simulink model "CAVE_MachE_Testing_testing_V2"  (R2024a)
settings: configuration reference "ConfigSetDesktopFixedStep" (kept outside this file)
PreLoadFcn:
  | VSS_BICYCLE=Simulink.Variant('Dual=0');
  | VSS_DUAL=Simulink.Variant('Dual=1');
  | Dual=1;
  | load('DriveCycle2.mat')
PostLoadFcn:
  | if any(exist('dsrtsu_mdlpostloadfcn', 'file') ~= 0), dsrtsu_mdlpostloadfcn('Execute', bdroot); end
InitFcn:
  | , if any(exist('rtifpga_mdlclblib', 'file') ~= 0), rtifpga_mdlclblib('Init', bdroot); end,
  | , if any(exist('dsmpb_private', 'file') ~= 0), dsmpb_private('dsmpb_mdlclblib', 'Init', bdroot); end,
  | load('DriveCycle2.mat')
model workspace (MAT data in the model file):
  Gas = 0.383333333333
undefined symbols (not defined in the file or in its folder): AccelCmd, ActTqLF_Nm_, ActTqLR_Nm_, ActTqRF_Nm_, ActTqRR_Nm_, BattChargeLimitMaxPwr, BattChargeLimitSocBpts, BattChargeLimitTbl, BattChrgCapcty, BattDischargeLimitSocBpts, BattDischargeLimitTbl, BattDischargeMaxPwr, BattNumCellsParallel, BattNumCellsSeries, BattOpenVoltCapBpts, BattOpenVoltTbl, BattResistSocBpts, BattResistTbl, BattResistTempBpts, BrakeMaxPrs, BrakeMaxTrq, ChassisDistCg2FrontAxle, ChassisDistCg2RearAxle, ChassisVehMass, CltchCmd, CoastDown, DecelCmd, DiffRatio, DiscIntNeverNeededParam, EnvGravCnst, EnvPrs, EnvTemp, FuelSpecificGrav, GearCmd, h, InitStates, lgSw, limitedMCT, MCT, MtrEffSpdBpts, MtrEffTbl, MtrEffTrqBpts, MtrPwrMax, MtrTrqMax, out_1, pMCT, RealSimPara, Ref_speed, Ref_time, SteeringCmd, SupvsryCtrlRegenBrkCutOffTbl, SupvsryCtrlRegenSpdBpts, TestScnrioCycleNum, US06, VEH
libraries: VSIGenLib x65, simulink x54, etargetslib x38, dsmpblib x24, vehdynlibtire x12, autolibshared x11, vehdynlibsuspension x7, vehdynlibtirecommon x7, autolibpowerinfoutils x6, autolibutils x5, autolibsharedcoupling x4, autolibmappedmotor x4
(part 3 of 17)

== system CAVE_MachE_Testing_testing_V2/RealSim2/ToRealSim/RealSim CreatBus ==
  In : Inport
  speedDesired : Inport  Port=2
  color : Inport  Port=3
  accelerationDesired : Inport  Port=4
  activeLaneChange : Inport  Port=5
  Bus Creator2 : BusCreator  Inputs=36  OutDataTypeStr=Bus: VehDataBus
  Bus Selector1 : BusSelector  OutputSignals=id,idLength,type,typeLength,vehicleClass,vehicleClassLength,speed,acceleration,positionX,positionY,positionZ,heading,color,linkId,linkIdLength,laneId,distanceTravel,speedDesired,accelerationDesired,hasPrecedingVehicle,precedingVehicleId,precedingVehicleIdLength,precedingVehicleDistance,precedingVehicleSpeed,signalLightId,signalLightIdLength,signalLightHeadId,signalLightDistance,signalLightColor,speedLimit,speedLimitNext,speedLimitChangeDistance,linkIdNext,linkIdNextLength,grade,activeLaneChange
  Terminator{4..7} (4 alike) : Terminator
  rgba2uint : Subsystem
  Out : Outport
  wires:
  Bus Creator2/1 -> Out/1
  rgba2uint/1(Out1) -> Bus Creator2/13  "color"
  color/1 -> rgba2uint/1(In1)  "color"
  accelerationDesired/1 -> Bus Creator2/19  "accelerationDesired"
  speedDesired/1 -> Bus Creator2/18  "speedDesired"
  activeLaneChange/1 -> Bus Creator2/36  "activeLaneChange"
  Bus Selector1/36 -> Terminator7/1  "<activeLaneChange>"
  Bus Selector1/35 -> Bus Creator2/35  "<grade>"
  Bus Selector1/34 -> Bus Creator2/34  "<linkIdNextLength>"
  Bus Selector1/33 -> Bus Creator2/33  "<linkIdNext>"
  Bus Selector1/32 -> Bus Creator2/32  "<speedLimitChangeDistance>"
  Bus Selector1/31 -> Bus Creator2/31  "<speedLimitNext>"
  Bus Selector1/30 -> Bus Creator2/30  "<speedLimit>"
  Bus Selector1/29 -> Bus Creator2/29  "<signalLightColor>"
  Bus Selector1/28 -> Bus Creator2/28  "<signalLightDistance>"
  Bus Selector1/27 -> Bus Creator2/27  "<signalLightHeadId>"
  Bus Selector1/26 -> Bus Creator2/26  "<signalLightIdLength>"
  Bus Selector1/25 -> Bus Creator2/25  "<signalLightId>"
  Bus Selector1/24 -> Bus Creator2/24  "<precedingVehicleSpeed>"
  Bus Selector1/23 -> Bus Creator2/23  "<precedingVehicleDistance>"
  Bus Selector1/22 -> Bus Creator2/22  "<precedingVehicleIdLength>"
  Bus Selector1/21 -> Bus Creator2/21  "<precedingVehicleId>"
  Bus Selector1/20 -> Bus Creator2/20  "<hasPrecedingVehicle>"
  Bus Selector1/19 -> Terminator6/1  "<accelerationDesired>"
  Bus Selector1/18 -> Terminator4/1  "<speedDesired>"
  Bus Selector1/17 -> Bus Creator2/17  "<distanceTravel>"
  Bus Selector1/16 -> Bus Creator2/16  "<laneId>"
  Bus Selector1/15 -> Bus Creator2/15  "<linkIdLength>"
  Bus Selector1/14 -> Bus Creator2/14  "<linkId>"
  Bus Selector1/13 -> Terminator5/1  "<color>"
  Bus Selector1/12 -> Bus Creator2/12  "<heading>"
  Bus Selector1/11 -> Bus Creator2/11  "<positionZ>"
  Bus Selector1/10 -> Bus Creator2/10  "<positionY>"
  Bus Selector1/9 -> Bus Creator2/9  "<positionX>"
  Bus Selector1/8 -> Bus Creator2/8  "<acceleration>"
  Bus Selector1/7 -> Bus Creator2/7  "<speed>"
  Bus Selector1/6 -> Bus Creator2/6  "<vehicleClassLength>"
  Bus Selector1/5 -> Bus Creator2/5  "<vehicleClass>"
  Bus Selector1/4 -> Bus Creator2/4  "<typeLength>"
  Bus Selector1/3 -> Bus Creator2/3  "<type>"
  Bus Selector1/2 -> Bus Creator2/2  "<idLength>"
  Bus Selector1/1 -> Bus Creator2/1  "<id>"
  In/1 -> Bus Selector1/1

== system CAVE_MachE_Testing_testing_V2/Vehicle Under Test1/Environment/Ground Feedback ==
  note: 1) Add Subsystem or Model blocks as valid variant choices.
      | 2) You cannot connect blocks at this level. At simulation, connectivity is automatically
      | determined, based on the active variant and port name matching.
  Friction : Inport
  Ground Z Level : Inport  Port=2
  3D Engine : Subsystem  VariantControl=1
  Constant : Subsystem  VariantControl=0
  Ground : Outport  VectorParamsAs1DForOutWhenUnconnected=off

== system CAVE_MachE_Testing_testing_V2/Vehicle Under Test1/Environment/Subsystem ==
  Grade : Inport
  Constant : Constant  Value=EnvPrs
  Constant1 : Constant  Value=EnvTemp
  Constant2 : Constant  Value=0
  Constant3 : Constant  Value=0
  Constant4 : Constant  Value=0
  Signal Specification : SignalSpecification  Unit=Pa
  Signal Specification1 : SignalSpecification  Unit=K
  Signal Specification2 : SignalSpecification  Unit=rad
  Signal Specification3 : SignalSpecification  Unit=m/s
  Signal Specification4 : SignalSpecification  Unit=m/s
  Signal Specification5 : SignalSpecification  Unit=m/s
  Vector Concatenate : Concatenate  NumInputs=3
  EnvPrs : Outport
  EnvTemp : Outport  Port=2
  WindVel : Outport  Port=3
  RoadGrade : Outport  Port=4
  wires:
  Signal Specification5/1 -> Vector Concatenate/3  "WindZ"
  Signal Specification4/1 -> Vector Concatenate/2  "WindY"
  Constant4/1 -> Signal Specification5/1
  Constant3/1 -> Signal Specification4/1
  Signal Specification3/1 -> Vector Concatenate/1  "WindX"
  Vector Concatenate/1 -> WindVel/1
  Signal Specification2/1 -> RoadGrade/1
  Signal Specification1/1 -> EnvTemp/1
  Signal Specification/1 -> EnvPrs/1
  Grade/1 -> Signal Specification2/1
  Constant1/1 -> Signal Specification1/1
  Constant2/1 -> Signal Specification3/1
  Constant/1 -> Signal Specification/1

== system CAVE_MachE_Testing_testing_V2/Vehicle Under Test1/Environment/Subsystem1 ==
  EnvPrs : Inport
  EnvTemp : Inport  Port=2
  WindVel : Inport  Port=3
  RoadGrade : Inport  Port=4
  GroundBus : Inport  Port=5
  Bus Creator : BusCreator  Inputs=5
  Env : Outport
  wires:
  GroundBus/1 -> Bus Creator/5  "GndBus"
  RoadGrade/1 -> Bus Creator/4  "RoadGrade"
  WindVel/1 -> Bus Creator/3  "WindVel"
  Bus Creator/1 -> Env/1  "Env"
  EnvTemp/1 -> Bus Creator/2  "EnvTemp"
  EnvPrs/1 -> Bus Creator/1  "EnvPrs"

== system CAVE_MachE_Testing_testing_V2/Vehicle Under Test1/Monitor/Calculate Fuel MPG ==
  Monitor : Inport
  Bus Selector : BusSelector  OutputSignals=Veh.Chassis.VehDist,Veh.Batt.EngPlant.FuellMassFlw
  Constant : Constant  Value=FuelSpecificGrav
  Density of Water : Gain  Gain=997
  Divide : Product  Inputs=*/
  Divide1 : Product  Inputs=*/
  Integrator : Integrator
  Saturation : Saturate  UpperLimit=inf  LowerLimit=1e-7
  Signal Specification : SignalSpecification  Unit=mi
  Signal Specification1 : SignalSpecification  Unit=m^3
  Signal Specification2 : SignalSpecification  Unit=gal
  Unit Conversion : UnitConversion
  Unit Conversion1 : UnitConversion
  FuelEconMPG : Outport
  wires:
  Signal Specification/1 -> Divide1/1  "VehDistMiles"
  Monitor/1 -> Bus Selector/1
  Signal Specification1/1 -> Unit Conversion1/1
  Constant/1 -> Density of Water/1
  Saturation/1 -> Divide1/2  "FuelVolume"
  Density of Water/1 -> Divide/2
  Integrator/1 -> Divide/1  "FuelMass"
  Bus Selector/2 -> Integrator/1  "<FuellMassFlw>"
  Bus Selector/1 -> Unit Conversion/1  "<VehDist>"
  Unit Conversion/1 -> Signal Specification/1
  Signal Specification2/1 -> Saturation/1
  Unit Conversion1/1 -> Signal Specification2/1
  Divide/1 -> Signal Specification1/1
  Divide1/1 -> FuelEconMPG/1  "FuelEconMPG"

== system CAVE_MachE_Testing_testing_V2/Vehicle Under Test1/Monitor/Calculate Powertrain Energy ==
  Monitor : Inport
  Bus Selector2 : BusSelector  OutputSignals=Veh.Diff.PwrInfo.PwrTrnsfrd.PwrTrnsfrd.PwrDriveshft
  Integrator : Integrator
  Signal Specification : SignalSpecification  Unit=J
  Signal Specification1 : SignalSpecification  Unit=kW*h
  Unit Conversion : UnitConversion
  TransEnrgyOutkWh : Outport
  wires:
  Bus Selector2/1 -> Integrator/1  "<PwrDriveshft>"
  Monitor/1 -> Bus Selector2/1
  Signal Specification1/1 -> TransEnrgyOutkWh/1
  Signal Specification/1 -> Unit Conversion/1
  Integrator/1 -> Signal Specification/1  "EnrgyTrans"
  Unit Conversion/1 -> Signal Specification1/1

== system CAVE_MachE_Testing_testing_V2/Vehicle Under Test1/Vehicle/Actuation and Outputs ==
  note: Driver Commands are [0,100] for both pedal and brake
  Driver Commands : Inport
  CarlaGBS : Inport  Port=2
  APP : Constant  Value=0
  AR_limit : Saturate  UpperLimit=65  LowerLimit=0
  BR_command_0to100 : Constant  Value=0
  BR_limit : Saturate  UpperLimit=70  LowerLimit=0
  Bus Creator : BusCreator  Inputs=2
  Bus Selector1 : BusSelector  OutputSignals=AccelPedalCmd
  Bus Selector3 : BusSelector  OutputSignals=BrakePedalCmd
  Constant : Constant  Value=0
  Constant1 : Constant  Value=0
  Demux : Demux  Outputs=3
  Gain : Gain  Gain=100
  Gain1 : Gain  Gain=100
  MOOG Brake Actuator : Subsystem
  Min threshold for Brake switch : Constant  Value=0
  Multiport Switch1 : MultiPortSwitch  Inputs=4  SaturateOnIntegerOverflow=off  InputSameDT=off
  Multiport Switch2 : MultiPortSwitch  Inputs=4  SaturateOnIntegerOverflow=off  InputSameDT=off
  Pedal Robot Control Selection : Constant  Value=2
  Relational Operator : RelationalOperator  Operator=>  OutDataTypeStr=boolean  InputSameDT=off
  Scope1 : Scope  NumInputPorts=2
  Vehicle Accel Pedal Voltage Output : Subsystem
  bped2br_N : Lookup_n-D  NumberOfTableDimensions=1  BreakpointsForDimension1=[0 0.1 0.2 100]  Table=[0 0 25 100]  InternalRulePriority=Speed  RndMeth=Simplest
  BrakeSwitch : Outport  VectorParamsAs1DForOutWhenUnconnected=off
  CAVE_Driver : Outport  Port=2
  tag scope: BrakeDriver=global, CarlaSteer=global, GasDriver=global
  wires:
  [BrakeDriver] -> Scope1/2
  [GasDriver] -> Scope1/1
  Demux/3 -> [CarlaSteer]
  Gain1/1 -> Multiport Switch2/4
  Gain/1 -> Multiport Switch1/4
  CarlaGBS/1 -> Demux/1
  Demux/2 -> Gain1/1
  Demux/1 -> Gain/1
  BR_limit/1 -> bped2br_N/1, Relational Operator/1, Bus Creator/2, [BrakeDriver]  "BrakePedalCmd_pct"
  AR_limit/1 -> Vehicle Accel Pedal Voltage Output/1(APP_pct), Bus Creator/1, [GasDriver]  "AccelPedalCmd_pct"
  Bus Creator/1 -> CAVE_Driver/1
  Constant1/1 -> Multiport Switch2/5
  Constant/1 -> Multiport Switch1/5
  Relational Operator/1 -> BrakeSwitch/1  "BrakeSwitch"
  Min threshold for Brake switch/1 -> Relational Operator/2
  bped2br_N/1 -> MOOG Brake Actuator/1(Brake Pedal command [%])
  Bus Selector3/1 -> Multiport Switch2/3  "<BrakePedalCmd>"
  BR_command_0to100/1 -> Multiport Switch2/2
  Pedal Robot Control Selection/1 -> Multiport Switch2/1, Multiport Switch1/1
  Driver Commands/1 -> Bus Selector1/1, Bus Selector3/1
  Multiport Switch2/1 -> BR_limit/1
  Bus Selector1/1 -> Multiport Switch1/3  "<AccelPedalCmd>"
  APP/1 -> Multiport Switch1/2
  Multiport Switch1/1 -> AR_limit/1

== system CAVE_MachE_Testing_testing_V2/Vehicle Under Test1/Vehicle/Battery ==
  Battery : Subsystem
  Subsystem1 : Subsystem
      mask Display: disp('')
  BattOut : PMIOPort  Side=Right
  BattOut1 : PMIOPort  Port=2  Side=Right
  Batt : Outport
  wires:
  Subsystem1/1(Batt) -> Batt/1
  Battery/3(BattVolt) -> Subsystem1/3(BattVolt)
  Battery/2(BattCurr) -> Subsystem1/2(BattCurr)
  Battery/1(BattSoc) -> Subsystem1/1(BattSoc)
  connections:
  BattOut/RConn1 -- Battery/RConn1
  Battery/RConn2 -- BattOut1/RConn1

== system CAVE_MachE_Testing_testing_V2/Vehicle Under Test1/Vehicle/Driver and Drive Cycle ==
  Veh speed feedback [kph] : Inport
  Veh speed cycle trigger : Inport  Port=2
  SUMO Veh speed Cmd Level : Inport  Port=3
  CarlaRef : Inport  Port=4
  1-D Lookup Table : Lookup_n-D  NumberOfTableDimensions=1  BreakpointsForDimension1=Ref_time  Table=Ref_speed  InternalRulePriority=Speed  RndMeth=Simplest
  Add : Sum
  Add1 : Sum  Inputs=+-
  Add2 : Sum
  Clock : Clock
  Clock1 : Clock
  CoastDown : Lookup_n-D  Commented=on  NumberOfTableDimensions=1  BreakpointsForDimension1=CoastDown.Time  Table=CoastDown.Speed  InternalRulePriority=Speed  RndMeth=Simplest
  Constant : Constant  Value=0
  Data Type Conversion11 : DataTypeConversion  OutDataTypeStr=double  SaturateOnIntegerOverflow=off  RndMeth=Floor  LockScale=on
  Demux : Demux  Outputs=3
  DriveCycleSelect : Constant  Commented=on
  Driver and PI with FF Control : Subsystem
  Gain : Gain  Gain=1/1.609
  Gain1 : Gain  Gain=1/1.609
  Gain2 : Gain  Gain=3.6
  Gain3 : Gain  Gain=3.6
  Get Cycle Clock Time : Subsystem
  MCT : Lookup_n-D  Commented=on  NumberOfTableDimensions=1  BreakpointsForDimension1=MCT.Time  Table=MCT.Speed  InternalRulePriority=Speed  RndMeth=Simplest
  ManSpd : Constant  Value=0
  ManSpdSel1 : Constant  Value=2
  Memory4 : Memory
  Multiport Switch : MultiPortSwitch  Commented=on  Inputs=5  SaturateOnIntegerOverflow=off  InputSameDT=off
  Multiport Switch1 : MultiPortSwitch  Inputs=4  SaturateOnIntegerOverflow=off  InputSameDT=off
  Rate Limiter : RateLimiter  RisingSlewLimit=5  FallingSlewLimit=-5  SampleTimeMode=inherited
  Scope : Scope  NumInputPorts=2
  Switch1 : Switch  Threshold=3  SaturateOnIntegerOverflow=off  InputSameDT=off
  Terminator{,1..3} (4 alike) : Terminator
  Terminator4 : Terminator  Commented=on
  US06 : Lookup_n-D  Commented=on  NumberOfTableDimensions=1  BreakpointsForDimension1=US06.Time  Table=US06.Speed  InternalRulePriority=Speed  RndMeth=Simplest
  US1 : Lookup_n-D  NumberOfTableDimensions=1  BreakpointsForDimension1=US06.Time  Table=US06.Speed  InternalRulePriority=Speed  RndMeth=Simplest
  driver look ahead seconds : Constant  Value=0.5
  limitedMCT : Lookup_n-D  Commented=on  NumberOfTableDimensions=1  BreakpointsForDimension1=limitedMCT.Time  Table=limitedMCT.Speed  InternalRulePriority=Speed  RndMeth=Simplest
  pMCT : Lookup_n-D  Commented=on  NumberOfTableDimensions=1  BreakpointsForDimension1=pMCT.Time  Table=pMCT.Speed  InternalRulePriority=Speed  RndMeth=Simplest
  DriverBus : Outport
  ManSpdSel : Outport  Port=2
  wires:
  US1/1 -> Rate Limiter/1
  Clock/1 -> Switch1/3
  Add2/1 -> Gain3/1
  Gain3/1 -> Multiport Switch1/4
  Memory4/1 -> Switch1/1
  Switch1/1 -> Memory4/1, Add1/2
  SUMO Veh speed Cmd Level/1 -> Add2/2
  Add1/1 -> 1-D Lookup Table/1  "tCycle"
  1-D Lookup Table/1 -> Add2/1
  ManSpdSel1/1 -> ManSpdSel/1, Multiport Switch1/1, Switch1/2
  Clock1/1 -> Add1/1, US1/1
  Constant/1 -> Multiport Switch1/5
  Demux/3 -> Terminator3/1
  Demux/2 -> Terminator2/1
  Demux/1 -> Gain2/1
  CarlaRef/1 -> Demux/1
  Gain2/1 -> Multiport Switch1/3
  Multiport Switch/1 -> Terminator4/1
  Rate Limiter/1 -> Multiport Switch1/2
  Multiport Switch1/1 -> Driver and PI with FF Control/2(Vehicle_SpdDmd_kph), Gain1/1, Scope/2  "RefSpd [km/hr]"
  Gain1/1 -> Terminator1/1  "Vehicle_SpdDmd_mph"
  Gain/1 -> Terminator/1  "Vehicle_Spd_mph"
  Veh speed feedback [kph]/1 -> [VehSpdKph]
  limitedMCT/1 -> Multiport Switch/6
  driver look ahead seconds/1 -> Add/1
  Get Cycle Clock Time/1(tCycle) -> Add/2
  Data Type Conversion11/1 -> Driver and PI with FF Control/1(Vehicle_Spd_kph), Scope/1, Gain/1  "Vehicle_Spd_kph"
  Driver and PI with FF Control/1(DriverBus) -> DriverBus/1
  [VehSpdKph] -> Data Type Conversion11/1
  DriveCycleSelect/1 -> Multiport Switch/1
  pMCT/1 -> Multiport Switch/3
  CoastDown/1 -> Multiport Switch/2
  Add/1 -> US06/1, MCT/1, limitedMCT/1, pMCT/1, CoastDown/1
  US06/1 -> Multiport Switch/4
  MCT/1 -> Multiport Switch/5
  Veh speed cycle trigger/1 -> Get Cycle Clock Time/1(Cycle Trigger)

== system CAVE_MachE_Testing_testing_V2/Vehicle Under Test1/Vehicle/From CAN ==
  BrakeSwitch : Inport
  Brake switch ource selection : Constant  Value=2
  Bus Creator1 : BusCreator  Inputs=2
  Demux : Demux  Outputs=1
  Ground : Ground
  Ground1 : Ground
  Multiport Switch1 : MultiPortSwitch  Inputs=2  SaturateOnIntegerOverflow=off  InputSameDT=off
  IO_Out : Outport
  wires:
  BrakeSwitch/1 -> Multiport Switch1/3
  Ground1/1 -> Multiport Switch1/2  "Brake switch from CAN"
  Brake switch ource selection/1 -> Multiport Switch1/1
  Ground/1 -> Demux/1
  Demux/1 -> Bus Creator1/1  "STEERING_ANGLE_DEG_CAN"
  Multiport Switch1/1 -> Bus Creator1/2  "BRAKE_LAMP_BOOL_CAN"
  Bus Creator1/1 -> IO_Out/1  "IO_Out"

== system CAVE_MachE_Testing_testing_V2/Vehicle Under Test1/Vehicle/Front Wheel Drive ==
  DrvShfTrq : Inport
  Omega : Inport  Port=2
  Ideal Diff : Subsystem  VariantControl=0
  Ideal Diff AWD : Subsystem  VariantControl=Choice
  Real Diff : Subsystem  VariantControl=1
  Diff : Outport  VectorParamsAs1DForOutWhenUnconnected=off
  AxlTrq : Outport  Port=2  VectorParamsAs1DForOutWhenUnconnected=off
  PropShaftSpd : Outport  Port=3  VectorParamsAs1DForOutWhenUnconnected=off
  PropShaftSpd1 : Outport  Port=4

== system CAVE_MachE_Testing_testing_V2/Vehicle Under Test1/Vehicle/Motor_F ==
  SupvsryCtrl : Inport
  MtrSpd : Inport  Port=2
  Bus Creator1 : BusCreator  Inputs=1
  Bus Creator2 : BusCreator  Inputs=4
  Bus Selector1 : BusSelector  OutputSignals=Volt
  Bus Selector2 : BusSelector  OutputSignals=MtrTrqCmd
  Bus Selector3 : BusSelector  OutputSignals=PwrInfo.PwrTrnsfrd.PwrMtr,PwrInfo.PwrTrnsfrd.PwrBus
  Mach-E Motor : autolibmappedmotor/Mapped Motor  port_config=Speed  param_by=Maximum torque and power  w_t=[ 0 375 750 800 ]  T_t=[0.09 0.08 0.07 0]  torque_max=800  power_max=358000  Tc=0.01  param_loss=Tabulated efficiency data  eff=100  w_eff=375  T_eff=0.08  Piron=0  Pbase=0  w_eff_bp=MtrEffSpdBpts.*pi/30  T_eff_bp=MtrEffTrqBpts  Temp_eff_bp=[233.15 293.15 373.15]  losses_table=[1 2;3 4]  losses_table_3d=cat(3,[1.49 1.67 2.21 3.10; 0.42 0.69 1.14 2.03; 0.06 0.24 0.78 1.68; 0.42 0.69 1.14 2.03; 1.49 1.67 2.21 3.10],[1.49 1.67 2.21 3.10; 0.42 0.69 1.14 2.03; 0.06 0.24 0.78 1.68; 0.42 0.69 1.14 2.03; 1.49 1.67 2.21 3.10],[1.49 1.67 2.21 3.10; 0.42 0.69 1.14 2.03; 0.06 0.24 0.78 1.68; 0.42 0.69 1.14 2.03; 1.49 1.67 2.21 3.10])  efficiency_table=MtrEffTbl*0.94  efficiency_table_3d=cat(3,[95 95 95 95; 95 95 95 95; 95 95 95 95; 95 95 95 95; 95 95 95 95],[95 95 95 95; 95 95 95 95; 95 95 95 95; 95 95 95 95; 95 95 95 95],[95 95 95 95; 95 95 95 95; 95 95 95 95; 95 95 95 95; 95 95 95 95])  J=5e-6  b=1e-5  omega_o=0  T_t_extended=[0 0.07 0.08 0.09 0.08 0.07 0]  w_t_extended=[-800 -750 -375 0 375 750 800]  KLossIron=0  KLossCopper=0  x_w_eff_vec=[-1047.1975511966 -942.477796076938 -837.758040957278 -733.038285837618 -628.318530717959 -523.598775598299 -418.879020478639 -314.159265358979 -285.714285713875 -209.43951023932 -104.71975511966 0 104.71975511966 209.43951023932 285.714285713875 314.159265358979 418.879020478639 523.598775598299 628.318530717959 733.038285837618 837.758040957278 942.477796076938 1047.1975511966]  x_T_eff_vec=[-360 -334.285714285714 -308.571428571429 -282.857142857143 -257.142857142857 -231.428571428571 -205.714285714286 -180 -154.285714285714 -128.571428571429 -102.857142857143 -77.1428571428572 -51.4285714285714 -25.7142857142857 0 25.7142857142857 51.4285714285714 77.1428571428572 102.857142857143 128.571428571429 154.285714285714 180 205.714285714286 231.428571428571 257.142857142857 282.857142857143 308.571428571429 334.285714285714 360]  x_tmp_eff_vec=[-0.09 -0.06 -0.03 0 0.03 0.06 0.09]  x_losses_mat=[54250.1517943165 50375.1409518653 46500.1301094142 42625.119266963 38750.1084245118 34875.0975820605 31000.0867396095 27125.0758971582 23250.065054707 19375.054212256 15500.0433698047 12629.4764797412 9803.55154311708 6774.11181875432 0 5412.5153431847 8293.80460547705 10921.9712596802 13550.1379138833 16937.6723923542 20325.2068708249 23712.7413492957 27100.2758277666 30487.8103062373 33875.3447847082 37262.879263179 40650.4137416499 44037.9482201206 47425.4826985915;44696.230836134 41503.6429192672 38311.0550024006 35118.4670855338 31925.8791686671 28733.2912518003 25540.7033349337 22348.115418067 19155.5275012002 15962.9395843336 12770.3516674669 9577.76375060014 6975.01951641212 6096.70063687888 0 4871.26380886623 6097.56206124747 8462.91205003029 11283.8827333737 14104.8534167172 16925.8241000605 19746.794783404 22567.7654667475 25388.7361500908 28209.7068334343 31030.6775167777 33851.6482001212 36672.6188834645 39493.589566808;36137.1105685043 33555.8883850397 30974.6662015752 28393.4440181105 25812.2218346459 23230.9996511813 20649.7774677168 18068.5552842522 15487.3331007875 12906.110917323 10324.8887338584 8513.56777831124 6200.01734792188 5419.28945500345 0 4330.01227454776 5420.05516555331 7522.58848891581 9220.12563933554 11525.1570491694 13830.1884590033 16135.2198688372 18440.2512786711 20745.2826885049 23050.3140983388 25355.3455081727 27660.3769180066 29965.4083278404 32270.4397376744;31619.9717474413 29361.4023369097 27102.8329263783 24844.2635158467 22585.6941053152 20327.1246947836 18068.5552842522 15809.9858737206 13551.4164631891 11292.8470526576 9034.27764212609 7449.37180602233 5425.01517943165 4741.87827312802 0 3788.76074022929 4742.54826985915 6582.26492780134 8067.6099344186 10084.5124180233 12101.4149016279 14118.3173852325 16135.2198688372 18152.1223524418 20169.0248360465 22185.9273196511 24202.8298032558 26219.7322868604 28236.6347704651;27102.8329263782 25166.9162887798 23230.9996511814 21295.0830135829 19359.1663759844 17423.249738386 15487.3331007876 13551.4164631891 11615.4998255906 9679.58318799226 8513.56777831124 6385.17583373343 4650.01301094141 4064.46709125259 0 3247.50920591082 4065.04137416498 5641.94136668686 7522.58848891582 8643.86778687709 10372.6413442524 12101.4149016279 13830.1884590033 15558.9620163787 17287.7355737541 19016.5091311295 20745.282688505 22474.0562458803 24202.8298032558;22585.6941053152 20972.4302406498 19359.1663759845 17745.9025113191 16132.6386466537 14519.3747819883 12906.110917323 11292.8470526576 9679.58318799221 8066.31932332688 7094.63981525937 5320.97986144452 3875.01084245118 3387.05590937716 0 2706.25767159235 3387.53447847082 4701.61780557238 6268.82374076318 7203.22315573091 8643.86778687704 10084.5124180232 11525.1570491694 12965.8016803156 14406.4463114618 15847.0909426079 17287.7355737541 18728.3802049003 20169.0248360465;19864.9914827262 18446.0635196743 17027.1355566225 15608.2075935706 14189.2796305187 12770.3516674668 11351.423704415 9932.4957413631 8513.56777831121 7094.63981525938 5675.71185220749 4256.78388915562 3100.00867396094 2709.64472750173 0 2165.00613727388 2710.02758277665 3761.29424445791 5015.05899261055 6268.82374076319 7522.58848891579 8776.35323706844 10030.1179852211 11283.8827333737 12537.6474815263 13791.412229679 15045.1769778316 16298.9417259842 17552.7064741369;20587.4582405459 19116.9255090783 17646.3927776108 16175.8600461432 12629.4764797412 11366.528831767 10103.581183793 8137.52276914747 6975.01951641211 5812.51626367679 4650.01301094142 3788.84294392236 2525.89529594824 2032.23354562629 0 1623.75460295541 2184.39425193603 3276.59137790406 4065.04137416499 5081.30171770625 6097.56206124746 7113.82240478872 8737.57700774416 9829.77413371214 10921.9712596802 13684.7775990372 14928.8482898587 16172.9189806802 17416.9896715018;18723.4042552922 17386.0182370571 16048.6322188219 14711.2462005868 11485.9634880614 10337.3671392553 9188.77079044916 8040.174441643 6891.57809283685 5742.98174403074 4594.38539522458 ...(+6536 chars)]  x_losses_mat_3d=[37.8947368421052 25.2631578947368 12.6315789473684 0 12 24 36;18.9473684210526 12.6315789473684 6.3157894736842 0 5.99999999999999 12 18;0 0 0 0 0 0 0;18 12 5.99999999999999 0 6.3157894736842 12.6315789473684 18.9473684210526;36 24 12 0 12.6315789473684 25.2631578947368 37.8947368421052]  CalLossMapData={}  CalLossWithTempMapData={}  aMode=aMode  RefBlkName='autolibmappedmotor/Mapped Motor'
  Mapped Motor : autolibmappedmotor/Mapped Motor  port_config=Speed  param_by=Maximum torque and power  w_t=[ 0 375 750 800 ]  T_t=[0.09 0.08 0.07 0]  torque_max=MtrTrqMax  power_max=MtrPwrMax  Tc=MtrTrqTimeCnst  param_loss=Tabulated efficiency data  eff=100  w_eff=375  T_eff=0.08  Piron=0  Pbase=0  w_eff_bp=MtrEffSpdBpts.*pi/30  T_eff_bp=MtrEffTrqBpts  Temp_eff_bp=[233.15 293.15 373.15]  losses_table=[1 2;3 4]  losses_table_3d=cat(3,[1.49 1.67 2.21 3.10; 0.42 0.69 1.14 2.03; 0.06 0.24 0.78 1.68; 0.42 0.69 1.14 2.03; 1.49 1.67 2.21 3.10],[1.49 1.67 2.21 3.10; 0.42 0.69 1.14 2.03; 0.06 0.24 0.78 1.68; 0.42 0.69 1.14 2.03; 1.49 1.67 2.21 3.10],[1.49 1.67 2.21 3.10; 0.42 0.69 1.14 2.03; 0.06 0.24 0.78 1.68; 0.42 0.69 1.14 2.03; 1.49 1.67 2.21 3.10])  efficiency_table=MtrEffTbl*0.94  efficiency_table_3d=cat(3,[95 95 95 95; 95 95 95 95; 95 95 95 95; 95 95 95 95; 95 95 95 95],[95 95 95 95; 95 95 95 95; 95 95 95 95; 95 95 95 95; 95 95 95 95],[95 95 95 95; 95 95 95 95; 95 95 95 95; 95 95 95 95; 95 95 95 95])  J=5e-6  b=1e-5  omega_o=0  T_t_extended=[0 0.07 0.08 0.09 0.08 0.07 0]  w_t_extended=[-800 -750 -375 0 375 750 800]  KLossIron=0  KLossCopper=0  x_w_eff_vec=[-1047.1975511966 -942.477796076938 -837.758040957278 -733.038285837618 -628.318530717959 -523.598775598299 -418.879020478639 -314.159265358979 -285.714285713875 -209.43951023932 -104.71975511966 0 104.71975511966 209.43951023932 285.714285713875 314.159265358979 418.879020478639 523.598775598299 628.318530717959 733.038285837618 837.758040957278 942.477796076938 1047.1975511966]  x_T_eff_vec=[-360 -334.285714285714 -308.571428571429 -282.857142857143 -257.142857142857 -231.428571428571 -205.714285714286 -180 -154.285714285714 -128.571428571429 -102.857142857143 -77.1428571428572 -51.4285714285714 -25.7142857142857 0 25.7142857142857 51.4285714285714 77.1428571428572 102.857142857143 128.571428571429 154.285714285714 180 205.714285714286 231.428571428571 257.142857142857 282.857142857143 308.571428571429 334.285714285714 360]  x_tmp_eff_vec=[-0.09 -0.06 -0.03 0 0.03 0.06 0.09]  x_losses_mat=[54250.1517943165 50375.1409518653 46500.1301094142 42625.119266963 38750.1084245118 34875.0975820605 31000.0867396095 27125.0758971582 23250.065054707 19375.054212256 15500.0433698047 12629.4764797412 9803.55154311708 6774.11181875432 0 5412.5153431847 8293.80460547705 10921.9712596802 13550.1379138833 16937.6723923542 20325.2068708249 23712.7413492957 27100.2758277666 30487.8103062373 33875.3447847082 37262.879263179 40650.4137416499 44037.9482201206 47425.4826985915;44696.230836134 41503.6429192672 38311.0550024006 35118.4670855338 31925.8791686671 28733.2912518003 25540.7033349337 22348.115418067 19155.5275012002 15962.9395843336 12770.3516674669 9577.76375060014 6975.01951641212 6096.70063687888 0 4871.26380886623 6097.56206124747 8462.91205003029 11283.8827333737 14104.8534167172 16925.8241000605 19746.794783404 22567.7654667475 25388.7361500908 28209.7068334343 31030.6775167777 33851.6482001212 36672.6188834645 39493.589566808;36137.1105685043 33555.8883850397 30974.6662015752 28393.4440181105 25812.2218346459 23230.9996511813 20649.7774677168 18068.5552842522 15487.3331007875 12906.110917323 10324.8887338584 8513.56777831124 6200.01734792188 5419.28945500345 0 4330.01227454776 5420.05516555331 7522.58848891581 9220.12563933554 11525.1570491694 13830.1884590033 16135.2198688372 18440.2512786711 20745.2826885049 23050.3140983388 25355.3455081727 27660.3769180066 29965.4083278404 32270.4397376744;31619.9717474413 29361.4023369097 27102.8329263783 24844.2635158467 22585.6941053152 20327.1246947836 18068.5552842522 15809.9858737206 13551.4164631891 11292.8470526576 9034.27764212609 7449.37180602233 5425.01517943165 4741.87827312802 0 3788.76074022929 4742.54826985915 6582.26492780134 8067.6099344186 10084.5124180233 12101.4149016279 14118.3173852325 16135.2198688372 18152.1223524418 20169.0248360465 22185.9273196511 24202.8298032558 26219.7322868604 28236.6347704651;27102.8329263782 25166.9162887798 23230.9996511814 21295.0830135829 19359.1663759844 17423.249738386 15487.3331007876 13551.4164631891 11615.4998255906 9679.58318799226 8513.56777831124 6385.17583373343 4650.01301094141 4064.46709125259 0 3247.50920591082 4065.04137416498 5641.94136668686 7522.58848891582 8643.86778687709 10372.6413442524 12101.4149016279 13830.1884590033 15558.9620163787 17287.7355737541 19016.5091311295 20745.282688505 22474.0562458803 24202.8298032558;22585.6941053152 20972.4302406498 19359.1663759845 17745.9025113191 16132.6386466537 14519.3747819883 12906.110917323 11292.8470526576 9679.58318799221 8066.31932332688 7094.63981525937 5320.97986144452 3875.01084245118 3387.05590937716 0 2706.25767159235 3387.53447847082 4701.61780557238 6268.82374076318 7203.22315573091 8643.86778687704 10084.5124180232 11525.1570491694 12965.8016803156 14406.4463114618 15847.0909426079 17287.7355737541 18728.3802049003 20169.0248360465;19864.9914827262 18446.0635196743 17027.1355566225 15608.2075935706 14189.2796305187 12770.3516674668 11351.423704415 9932.4957413631 8513.56777831121 7094.63981525938 5675.71185220749 4256.78388915562 3100.00867396094 2709.64472750173 0 2165.00613727388 2710.02758277665 3761.29424445791 5015.05899261055 6268.82374076319 7522.58848891579 8776.35323706844 10030.1179852211 11283.8827333737 12537.6474815263 13791.412229679 15045.1769778316 16298.9417259842 17552.7064741369;20587.4582405459 19116.9255090783 17646.3927776108 16175.8600461432 12629.4764797412 11366.528831767 10103.581183793 8137.52276914747 6975.01951641211 5812.51626367679 4650.01301094142 3788.84294392236 2525.89529594824 2032.23354562629 0 1623.75460295541 2184.39425193603 3276.59137790406 4065.04137416499 5081.30171770625 6097.56206124746 7113.82240478872 8737.57700774416 9829.77413371214 10921.9712596802 13684.7775990372 14928.8482898587 16172.9189806802 17416.9896715018;18723.4042552922 17386.0182370571 16048.6322188219 14711.2462005868 11485.9634880614 10337.3671392553 9188.77079044916 8040.174441643 6891.57809283685 5742.98174403074 4594.38539522458 ...(+6536 chars)]  x_losses_mat_3d=[37.8947368421052 25.2631578947368 12.6315789473684 0 12 24 36;18.9473684210526 12.6315789473684 6.3157894736842 0 5.99999999999999 12 18;0 0 0 0 0 0 0;18 12 5.99999999999999 0 6.3157894736842 12.6315789473684 18.9473684210526;36 24 12 0 12.6315789473684 25.2631578947368 37.8947368421052]  CalLossMapData={}  CalLossWithTempMapData={}  aMode=aMode  RefBlkName='autolibmappedmotor/Mapped Motor'
  Memory : Memory
  Mux{,1..3} (4 alike) : Mux  Inputs=1
  Scope : Scope
  To Workspace : ToWorkspace  VariableName=MtrTrq_F_Mache  SaveFormat=Structure With Time  SampleTime=-1
  Two-Way Connection1 : TwoWayConnection
  Batt : PMIOPort  Side=Left
  Mtr : Outport
  MtrTrq : Outport  Port=2
  wires:
  Mach-E Motor/3 -> Mux/1, MtrTrq/1, To Workspace/1  "Trq"
  Mach-E Motor/2 -> Memory/1  "Curr"
  Bus Creator1/1 -> Two-Way Connection1/1
  Mach-E Motor/1 -> Bus Selector3/1
  SupvsryCtrl/1 -> Bus Selector2/1
  Two-Way Connection1/1 -> Bus Selector1/1
  Bus Selector1/1 -> Mach-E Motor/1  "<Volt>"
  Bus Selector2/1 -> Scope/1, Mach-E Motor/3  "<MtrTrqCmd>"
  Mux/1 -> Bus Creator2/2  "MtrTrq"
  Bus Creator2/1 -> Mtr/1
  Mux2/1 -> Bus Creator2/3  "MtrMechPwr"
  Bus Selector3/1 -> Mux2/1  "<PwrMtr>"
  Mux1/1 -> Bus Creator2/1  "MtrSpd"
  Bus Selector3/2 -> Mux3/1  "<PwrBus>"
  Mux3/1 -> Bus Creator2/4  "MtrElecPwr"
  Memory/1 -> Bus Creator1/1  "Curr"
  MtrSpd/1 -> Mach-E Motor/2, Mux1/1
  connections:
  Batt/RConn1 -- Two-Way Connection1/RConn1
